simulink model "Citation_2017a"  (R2017a)
settings: Solver=ode5  StartTime=0.0  StopTime=inf  FixedStep=0.01  RelTol=1e-3  EnableMultiTasking=on
InitFcn:
  | initcit
values from neighbouring files (symbols this model uses):
  aeroinit = [dp_ini;inicoef('CX0');inicoef('CXa');inicoef('CXa2');inicoef('CXq')     ;inicoef('CXde');inicoef('CY0');inicoef('CYB');inicoef('CYp');inicoef('CYr')     ;inicoef('CYda');inicoef('CYdr');inicoef('CZ0');inicoef('CZa');inicoef('CZq')     ;inicoef('CZde');inicoef('Cl0');inicoef('ClB');inicoef('Clp');inicoef('Clr')     ;inicoef('Clda');inicoef('Cldr');inicoef('Cm0');inicoef('Cma');inicoef('Cmq')     ; ...(+113 chars)    [initcit.m]
  Clda_thresh = 3.410e-2/2    (= 0.01705)    [initcit.m]
  h_l_old = zeros(6,sample_size)    [initcit.m]
  h_m_old = zeros(4,sample_size)    [initcit.m]
  h_n_old = zeros(6,sample_size)    [initcit.m]
  h_X_old = zeros(5,sample_size)    [initcit.m]
  h_Y_old = zeros(6,sample_size)    [initcit.m]
  h_Z_old = zeros(4,sample_size)    [initcit.m]
  I = [massinit(5),0, -massinit(8);0, massinit(6),0;-massinit(8),0, massinit(7)]    [initcit.m]
  p_l = [inicoef('Cl0');inicoef('ClB');inicoef('Clp');inicoef('Clr')     ;inicoef('Clda');inicoef('Cldr')].*ones(6,sample_size)    [initcit.m]
  p_m = [inicoef('Cm0');inicoef('Cma');inicoef('Cmq')     ;inicoef('Cmde')].*ones(4,sample_size)    [initcit.m]
  p_n = [inicoef('Cn0');inicoef('CnB');inicoef('Cnp');inicoef('Cnr')     ;inicoef('Cnda');inicoef('Cndr')].*ones(6,sample_size)    [initcit.m]
  p_X = [inicoef('CX0');inicoef('CXa');inicoef('CXa2');inicoef('CXq')     ;inicoef('CXde')].*ones(5,sample_size)    [initcit.m]
  p_Y = [inicoef('CY0');inicoef('CYB');inicoef('CYp');inicoef('CYr')     ;inicoef('CYda');inicoef('CYdr')].*ones(6,sample_size)    [initcit.m]
  p_Z = [inicoef('CZ0');inicoef('CZa');inicoef('CZq')     ;inicoef('CZde')].*ones(4,sample_size)    [initcit.m]
  Pcov_l = 10000*eye(6)    [initcit.m]
  Pcov_m = 10000*eye(4)    [initcit.m]
  Pcov_n = 10000*eye(6)    [initcit.m]
  Pcov_X = 10000*eye(5)    [initcit.m]
  Pcov_Y = 10000*eye(6)    [initcit.m]
  Pcov_Z = 10000*eye(4)    [initcit.m]
  replay = 0    [initcit.m]
  T0 = 288.15    [rho_test.m]
  timeend = inputsim.data{1}.Values.Time(end)    [initcit.m]
  Vw915 = 0    [initcit.m]
  winddir = 45*(pi/180)    (= 0.785398163397)    [initcit.m]
  x0 = []    [cessnac550_3d_sfnc.m]    (also in sfunxyauto.m)
  y_l = zeros(1,sample_size)    [initcit.m]
  y_l_est_old = zeros(size(y_l))    [initcit.m]
  y_m = zeros(1,sample_size)    [initcit.m]
  y_m_est_old = zeros(size(y_m))    [initcit.m]
  y_n = zeros(1,sample_size)    [initcit.m]
  y_n_est_old = zeros(size(y_n))    [initcit.m]
  y_X = zeros(1,sample_size)    [initcit.m]
  y_X_est_old = zeros(size(y_X))    [initcit.m]
  y_Y = zeros(1,sample_size)    [initcit.m]
  y_Y_est_old = zeros(size(y_Y))    [initcit.m]
  y_Z = zeros(1,sample_size)    [initcit.m]
  y_Z_est_old = zeros(size(y_Z))    [initcit.m]
undefined symbols (not defined in the file or in its folder): chord, cv1, cv2, cv3, cv4, deltagmax1, deltagmax2, deltagmax3, deltagmax4, Deng, ealphag, ealphas, g0, hDME, hGS, kt1, kt2, kt3, lh, massinit, matbuaf, matdaf, matdam, matdbbf, matdeaf, matdgaf, matdqaf, matduaf, matdwaw, matedhr, mateif, matelhr, matemhr, matemv1, matemv2, matemve, matetam, mateuaf, matfaaf, matfaxl, matff, matibaf, matibmh, matipaf, matipmh, matiraf, matiuaf, matiwaf, matlaf, matlam, matleaf, matleam, matlgaf, matlqaf, matluaf, matmaaf, matmaam, matmaf, matmam, matmbbf ... (+74)
undefined symbols (not defined in the file): matibb
libraries: simulink x13, templibrary x6, vrlib x1
(part 6 of 7)

== system Citation_2017a/Cessna Citation 500/Citation model DASMAT/AIRCRAFT MODEL/AFM/Aeromod/SubSystem/model/CYCAL ==
  in_1 : Inport
  Abs : Abs  SaturateOnIntegerOverflow=on
  CY : Sum  Inputs=+++++  SaturateOnIntegerOverflow=on  InputSameDT=on  OutDataTypeStr=Inherit: Same as first input
  CY/ BETA : Sum  SaturateOnIntegerOverflow=on  InputSameDT=on  OutDataTypeStr=Inherit: Same as first input
  CYBAB : Lookup2D  RowIndex=matybab(2:5,1)  ColumnIndex=matybab(1,2:5)  Table=matybab(2:5,2:5)  SaturateOnIntegerOverflow=on  InputSameDT=on
  CYBAF : Lookup2D  RowIndex=matybaf(2:3,1)  ColumnIndex=matybaf(1,2:3)  Table=matybaf(2:3,2:3)  SaturateOnIntegerOverflow=on  InputSameDT=on
  CYBETA : Product  SaturateOnIntegerOverflow=on  InputSameDT=on  OutDataTypeStr=Inherit: Same as first input
  CYBUAF : Lookup2D  RowIndex=matbuaf(2:3,1)  ColumnIndex=matbuaf(1,2:3)  Table=matbuaf(2:3,2:3)  SaturateOnIntegerOverflow=on  InputSameDT=on
  CYBUC : Product  SaturateOnIntegerOverflow=on  InputSameDT=on  OutDataTypeStr=Inherit: Same as first input
  CYDA : Product  SaturateOnIntegerOverflow=on  InputSameDT=on  OutDataTypeStr=Inherit: Same as first input
  CYDR : Product  Inputs=3  SaturateOnIntegerOverflow=on  InputSameDT=on  OutDataTypeStr=Inherit: Same as first input
  CYGUST : Mux  Inputs=8
  CYR : Product  SaturateOnIntegerOverflow=on  InputSameDT=on  OutDataTypeStr=Inherit: Same as first input
  CYRAF : Lookup2D  RowIndex=matyraf(2:3,1)  ColumnIndex=matyraf(1,2:3)  Table=matyraf(2:3,2:3)  SaturateOnIntegerOverflow=on  InputSameDT=on
  CYRUAF : Lookup2D  RowIndex=matyuaf(2:3,1)  ColumnIndex=matyuaf(1,2:3)  Table=matyuaf(2:3,2:3)  SaturateOnIntegerOverflow=on  InputSameDT=on
  CYWAF : Lookup2D  RowIndex=matywaf(2:3,1)  ColumnIndex=matywaf(1,2:3)  Table=matywaf(2:3,2:3)  SaturateOnIntegerOverflow=on  InputSameDT=on
  Demux : Demux  Outputs=[1 1 1 1 1 1 1 1 1 1 1 1 1 1 1 1 1 1]
  KUUT : Lookup  InputValues=matuut(1,:)  Table=matuut(2,:)  SaturateOnIntegerOverflow=on
  LSFACT : Subsystem
  Prod : Product  SaturateOnIntegerOverflow=on  InputSameDT=on  OutDataTypeStr=Inherit: Same as first input
  Sum : Sum  SaturateOnIntegerOverflow=on  InputSameDT=on  OutDataTypeStr=Inherit: Same as first input
  Terminator_{1..11} (11 alike) : Terminator
  zero : Constant  Value=0
  out_1 : Outport
  out_2 : Outport  Port=2
  wires:
  Demux/18 -> Terminator_11/1
  Demux/17 -> Terminator_10/1
  Demux/16 -> Terminator_9/1
  Demux/13 -> Terminator_8/1
  Demux/12 -> Terminator_7/1
  Demux/11 -> Terminator_6/1
  Demux/8 -> Terminator_5/1
  Demux/7 -> Terminator_4/1
  Demux/6 -> Terminator_3/1
  Demux/2 -> Terminator_2/1
  Demux/1 -> Terminator_1/1
  CY/ BETA/1 -> CYGUST/3
  CYBUAF/1 -> Prod/1
  CYBUC/1 -> CY/5
  CYR/1 -> CY/4
  CYBETA/1 -> CY/1
  CYRAF/1 -> CYR/2
  CYWAF/1 -> CYDA/2
  CYBAB/1 -> Sum/2
  CYBAF/1 -> Sum/1
  Abs/1 -> CYBAB/1
  CY/1 -> out_1/1
  KUUT/1 -> Prod/2
  Demux/14 -> CYBAF/1, CYRUAF/1, CYRAF/1, CYBUAF/1, CYWAF/1
  Demux/5 -> CYBETA/1, Abs/1, CYBUC/1
  Demux/4 -> CYBAF/2, CYWAF/2, CYRAF/2, CYBUAF/2, CYRUAF/2, CYBAB/2
  CYGUST/1 -> out_2/1
  zero/1 -> CYGUST/2, CYGUST/7, CYGUST/8, CYGUST/6, CYGUST/5, CYGUST/4, CYGUST/1
  in_1/1 -> Demux/1
  CYRUAF/1 -> CYDR/2
  Demux/10 -> CYDR/1, LSFACT/1(deltar)
  Sum/1 -> CY/ BETA/1, CYBETA/2
  Prod/1 -> CY/ BETA/2, CYBUC/2
  CYDA/1 -> CY/2
  CYDR/1 -> CY/3
  Demux/3 -> CYR/1
  Demux/15 -> KUUT/1
  Demux/9 -> CYDA/1
  LSFACT/1(LSFACT) -> CYDR/3

== system Citation_2017a/Cessna Citation 500/Citation model DASMAT/AIRCRAFT MODEL/EFM/Engmod/Citation eng_mod/Subsystem1/JT15 Dynamic ==
  In1 : Inport
  Demux : Demux  Outputs=32
  Mux : Mux  Inputs=11
  Subsystem : Subsystem
  Out1 : Outport
  wires:
  Demux/32 -> Subsystem/32(Deng)
  Demux/31 -> Subsystem/31(VIAS)
  Demux/30 -> Subsystem/30(VCAS)
  Demux/29 -> Subsystem/29(VEAS)
  Demux/28 -> Subsystem/28(temptot)
  Demux/27 -> Subsystem/27(ptot)
  Demux/26 -> Subsystem/26(qrel)
  Demux/25 -> Subsystem/25(qc)
  Demux/24 -> Subsystem/24(Reynl)
  Demux/23 -> Subsystem/23(qdyn)
  Demux/22 -> Subsystem/22(Mach)
  Demux/21 -> Subsystem/21(Vsound)
  Demux/20 -> Subsystem/20(Hgeopot)
  Demux/19 -> Subsystem/19(hradio)
  Demux/18 -> Subsystem/18(hpress)
  Demux/17 -> Subsystem/17(grav)
  Demux/16 -> Subsystem/16(temp)
  Demux/15 -> Subsystem/15(rho)
  Demux/14 -> Subsystem/14(pstat)
  Demux/13 -> Subsystem/13(ut)
  Demux/12 -> Subsystem/12(ye)
  Demux/11 -> Subsystem/11(xe)
  Demux/10 -> Subsystem/10(he)
  Demux/9 -> Subsystem/9(psi)
  Demux/8 -> Subsystem/8(theta)
  Demux/7 -> Subsystem/7(phi)
  Demux/6 -> Subsystem/6(beta)
  Demux/5 -> Subsystem/5(alpha)
  Demux/4 -> Subsystem/4(VTAS)
  Demux/3 -> Subsystem/3(rbody)
  Demux/2 -> Subsystem/2(qbody)
  Demux/1 -> Subsystem/1(pbody)
  Subsystem/2(FF) -> Mux/2
  Subsystem/3(N1) -> Mux/3
  Subsystem/4(N2) -> Mux/4
  Subsystem/5(N1c) -> Mux/5
  Subsystem/6(N2c) -> Mux/6
  Subsystem/7(WT) -> Mux/7
  Subsystem/8(ITT) -> Mux/8
  Subsystem/9(EGT) -> Mux/9
  Subsystem/10(OILT) -> Mux/10
  Subsystem/11(OILP) -> Mux/11
  Subsystem/1(Tn) -> Mux/1
  In1/1 -> Demux/1
  Mux/1 -> Out1/1

== system Citation_2017a/Cessna Citation 500/Citation model DASMAT/AIRCRAFT MODEL/EFM/Engmod/Citation eng_mod/Subsystem1/JT15 Dynamic1 ==
  In1 : Inport
  Demux : Demux  Outputs=32
  Mux : Mux  Inputs=11
  Subsystem : Subsystem
  Out1 : Outport
  wires:
  Demux/32 -> Subsystem/32(Deng)
  Demux/31 -> Subsystem/31(VIAS)
  Demux/30 -> Subsystem/30(VCAS)
  Demux/29 -> Subsystem/29(VEAS)
  Demux/28 -> Subsystem/28(temptot)
  Demux/27 -> Subsystem/27(ptot)
  Demux/26 -> Subsystem/26(qrel)
  Demux/25 -> Subsystem/25(qc)
  Demux/24 -> Subsystem/24(Reynl)
  Demux/23 -> Subsystem/23(qdyn)
  Demux/22 -> Subsystem/22(Mach)
  Demux/21 -> Subsystem/21(Vsound)
  Demux/20 -> Subsystem/20(Hgeopot)
  Demux/19 -> Subsystem/19(hradio)
  Demux/18 -> Subsystem/18(hpress)
  Demux/17 -> Subsystem/17(grav)
  Demux/16 -> Subsystem/16(temp)
  Demux/15 -> Subsystem/15(rho)
  Demux/14 -> Subsystem/14(pstat)
  Demux/13 -> Subsystem/13(ut)
  Demux/12 -> Subsystem/12(ye)
  Demux/11 -> Subsystem/11(xe)
  Demux/10 -> Subsystem/10(he)
  Demux/9 -> Subsystem/9(psi)
  Demux/8 -> Subsystem/8(theta)
  Demux/7 -> Subsystem/7(phi)
  Demux/6 -> Subsystem/6(beta)
  Demux/5 -> Subsystem/5(alpha)
  Demux/4 -> Subsystem/4(VTAS)
  Demux/3 -> Subsystem/3(rbody)
  Demux/2 -> Subsystem/2(qbody)
  Demux/1 -> Subsystem/1(pbody)
  Subsystem/2(FF) -> Mux/2
  Subsystem/3(N1) -> Mux/3
  Subsystem/4(N2) -> Mux/4
  Subsystem/5(N1c) -> Mux/5
  Subsystem/6(N2c) -> Mux/6
  Subsystem/7(WT) -> Mux/7
  Subsystem/8(ITT) -> Mux/8
  Subsystem/9(EGT) -> Mux/9
  Subsystem/10(OILT) -> Mux/10
  Subsystem/11(OILP) -> Mux/11
  Subsystem/1(Tn) -> Mux/1
  In1/1 -> Demux/1
  Mux/1 -> Out1/1

== system Citation_2017a/Cessna Citation 500/Citation model DASMAT/AIRCRAFT MODEL/AFM/Aeromod/SubSystem/model/CDCAL/KBASD ==
  hcg : Inport
  deltaf : Inport  Port=2
  VEAS : Inport  Port=3
  Constant : Constant
  Fcn : Fcn  Expr=0.2-u[1]
  Fcn1 : Fcn  Expr=u[2]*(u[1]*180/pi-15)*0.04*(100-u[3])/30
  Fcn2 : Fcn  Expr=1-0.6*u[1]
  KGEDHR : Lookup  InputValues=matedhr(1,:)  Table=matedhr(2,:)  SaturateOnIntegerOverflow=on
  Mux : Mux  Inputs=3
  Sat : Saturate  UpperLimit=1  LowerLimit=0
  Switch : Switch  SaturateOnIntegerOverflow=on  InputSameDT=on
  KBASD : Outport
  wires:
  KGEDHR/1 -> Mux/2
  deltaf/1 -> Mux/1, Fcn/1
  Fcn/1 -> Switch/2
  Constant/1 -> Switch/1
  Switch/1 -> KBASD/1
  VEAS/1 -> Mux/3
  hcg/1 -> KGEDHR/1
  Mux/1 -> Fcn1/1
  Sat/1 -> Fcn2/1
  Fcn1/1 -> Sat/1
  Fcn2/1 -> Switch/3

== system Citation_2017a/Cessna Citation 500/Citation model DASMAT/AIRCRAFT MODEL/AFM/Aeromod/SubSystem/model/CLCAL/CLGEAF ==
  alpha : Inport
  deltaf : Inport  Port=2
  Prod : Product  SaturateOnIntegerOverflow=on  InputSameDT=on  OutDataTypeStr=Inherit: Same as first input
  Sat : Saturate  UpperLimit=0.04  LowerLimit=-inf
  Sum : Sum  SaturateOnIntegerOverflow=on  InputSameDT=on  OutDataTypeStr=Inherit: Same as first input
  VDOMMYR37 : Lookup  InputValues=vdommyr37(1,:)  Table=vdommyr37(2,:)  SaturateOnIntegerOverflow=on
  VDOMMYR40 : Gain  Gain=1.6  SaturateOnIntegerOverflow=on  OutDataTypeStr=Inherit: Same as input  ParamDataTypeStr=Inherit: Same as input
  rad2deg : Gain  Gain=(180/pi)  SaturateOnIntegerOverflow=on  OutDataTypeStr=Inherit: Same as input  ParamDataTypeStr=Inherit: Same as input
  CLGEAF : Outport
  wires:
  VDOMMYR37/1 -> VDOMMYR40/1, Prod/2
  rad2deg/1 -> Prod/1
  Sat/1 -> rad2deg/1
  alpha/1 -> Sat/1
  deltaf/1 -> VDOMMYR37/1
  VDOMMYR40/1 -> Sum/2
  Prod/1 -> Sum/1
  Sum/1 -> CLGEAF/1

== system Citation_2017a/Cessna Citation 500/Citation model DASMAT/AIRCRAFT MODEL/AFM/Aeromod/SubSystem/model/CLCAL/SP0 ==
  deltae : Inport
  Abs : Abs  SaturateOnIntegerOverflow=on
  Fcn : Fcn  Expr=(0.087+0.25*(u[1]-0.087))/(u[1]+1e-11)
  Prod : Product  SaturateOnIntegerOverflow=on  InputSameDT=on  OutDataTypeStr=Inherit: Same as first input
  Sat : Saturate  UpperLimit=1  LowerLimit=-inf
  SP0 : Outport
  wires:
  deltae/1 -> Prod/1, Abs/1
  Sat/1 -> Prod/2
  Fcn/1 -> Sat/1
  Abs/1 -> Fcn/1
  Prod/1 -> SP0/1

== system Citation_2017a/Cessna Citation 500/Citation model DASMAT/AIRCRAFT MODEL/AFM/Aeromod/SubSystem/model/CLLCAL/CIBAB ==
  note: 02-11-2000
      | Modified by A. R. Veldhuijzen
      | sftable3.m was replaced with table3.dll
      | X and Y are exchanged in this Mathworks implementation
  x0 : Inport
  y0 : Inport  Port=2
  z0 : Inport  Port=3
  Mux : Mux  Inputs=3
  S-function : S-Function  FunctionName=table3  Parameters=yindex, xindex ,zindex, table  SFunctionDeploymentMode=off  EnableBusSupport=off
  out_1 : Outport
  wires:
  z0/1 -> Mux/3
  y0/1 -> Mux/1
  x0/1 -> Mux/2
  Mux/1 -> S-function/1
  S-function/1 -> out_1/1

== system Citation_2017a/Cessna Citation 500/Citation model DASMAT/AIRCRAFT MODEL/AFM/Aeromod/SubSystem/model/CLLCAL/LFACT ==
  hcg : Inport
  Sat : Saturate  UpperLimit=1  LowerLimit=0
  hrunway : Fcn  Expr=1-(u[1]-1)/30
  LFACT : Outport
  wires:
  Sat/1 -> LFACT/1
  hcg/1 -> hrunway/1
  hrunway/1 -> Sat/1

== system Citation_2017a/Cessna Citation 500/Citation model DASMAT/AIRCRAFT MODEL/AFM/Aeromod/SubSystem/model/CMCAL/EALPHA ==
  alpha : Inport
  deltaf : Inport  Port=2
  Fcn : Fcn  Expr=1-u[1]*u[2]
  Mux : Mux  Inputs=2
  Sat : Saturate  UpperLimit=1  LowerLimit=0
  Sum : Sum  Inputs=+-  SaturateOnIntegerOverflow=on  InputSameDT=on  OutDataTypeStr=Inherit: Same as first input
  ealphag : Lookup  InputValues=ealphag(1,:)  Table=ealphag(2,:)  SaturateOnIntegerOverflow=on
  ealphas : Lookup  InputValues=ealphas(1,:)  Table=ealphas(2,:)  SaturateOnIntegerOverflow=on
  EALPHA : Outport
  wires:
  deltaf/1 -> ealphag/1, ealphas/1
  alpha/1 -> Sum/1
  Mux/1 -> Fcn/1
  ealphag/1 -> Mux/2
  ealphas/1 -> Sum/2
  Sum/1 -> Mux/1
  Fcn/1 -> Sat/1
  Sat/1 -> EALPHA/1

== system Citation_2017a/Cessna Citation 500/Citation model DASMAT/AIRCRAFT MODEL/AFM/Aeromod/SubSystem/model/CMCAL/LFCMEGAF ==
  alpha : Inport
  Abs : Abs  SaturateOnIntegerOverflow=on
  Fcn : Fcn  Expr=1-5*u[1]
  Neg : Gain  Gain=-1  SaturateOnIntegerOverflow=on  OutDataTypeStr=Inherit: Same as input  ParamDataTypeStr=Inherit: Same as input
  Sat : Saturate  UpperLimit=inf  LowerLimit=0.25
  LFCMEGAF : Outport
  wires:
  Fcn/1 -> Sat/1
  alpha/1 -> Abs/1
  Abs/1 -> Fcn/1
  Sat/1 -> Neg/1
  Neg/1 -> LFCMEGAF/1

== system Citation_2017a/Cessna Citation 500/Citation model DASMAT/AIRCRAFT MODEL/AFM/Aeromod/SubSystem/model/CYCAL/LSFACT ==
  deltar : Inport
  Abs : Abs  SaturateOnIntegerOverflow=on
  Fcn : Fcn  Expr=0.06981/u[1]+2*(u[1]-0.06981)
  Sat : Saturate  UpperLimit=inf  LowerLimit=0.06981
  LSFACT : Outport
  wires:
  deltar/1 -> Abs/1
  Abs/1 -> Sat/1
  Sat/1 -> Fcn/1
  Fcn/1 -> LSFACT/1

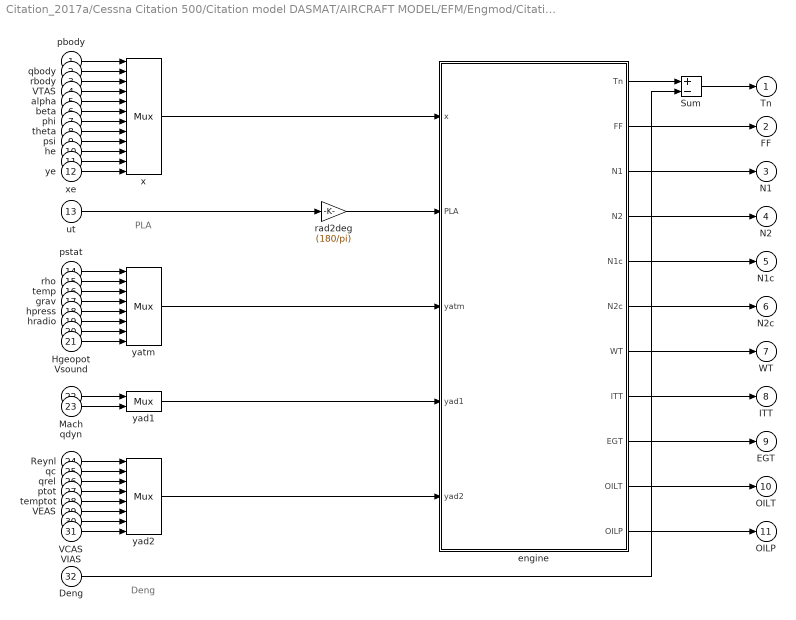
== system Citation_2017a/Cessna Citation 500/Citation model DASMAT/AIRCRAFT MODEL/EFM/Engmod/Citation eng_mod/Subsystem1/JT15 Dynamic/Subsystem ==
  note: Deng
  note: PLA
  pbody : Inport
  qbody : Inport  Port=2
  rbody : Inport  Port=3
  VTAS : Inport  Port=4
  alpha : Inport  Port=5
  beta : Inport  Port=6
  phi : Inport  Port=7
  theta : Inport  Port=8
  psi : Inport  Port=9
  he : Inport  Port=10
  xe : Inport  Port=11
  ye : Inport  Port=12
  ut : Inport  Port=13
  pstat : Inport  Port=14
  rho : Inport  Port=15
  temp : Inport  Port=16
  grav : Inport  Port=17
  hpress : Inport  Port=18
  hradio : Inport  Port=19
  Hgeopot : Inport  Port=20
  Vsound : Inport  Port=21
  Mach : Inport  Port=22
  qdyn : Inport  Port=23
  Reynl : Inport  Port=24
  qc : Inport  Port=25
  qrel : Inport  Port=26
  ptot : Inport  Port=27
  temptot : Inport  Port=28
  VEAS : Inport  Port=29
  VCAS : Inport  Port=30
  VIAS : Inport  Port=31
  Deng : Inport  Port=32
  Sum : Sum  Inputs=+-  SaturateOnIntegerOverflow=on  InputSameDT=on  OutDataTypeStr=Inherit: Same as first input
  engine : Subsystem
  rad2deg : Gain  Gain=(180/pi)  SaturateOnIntegerOverflow=on  OutDataTypeStr=Inherit: Same as input  ParamDataTypeStr=Inherit: Same as input
  x : Mux  Inputs=12
  yad1 : Mux  Inputs=2
  yad2 : Mux  Inputs=8
  yatm : Mux  Inputs=8
  Tn : Outport
  FF : Outport  Port=2
  N1 : Outport  Port=3
  N2 : Outport  Port=4
  N1c : Outport  Port=5
  N2c : Outport  Port=6
  WT : Outport  Port=7
  ITT : Outport  Port=8
  EGT : Outport  Port=9
  OILT : Outport  Port=10
  OILP : Outport  Port=11
  wires:
  Deng/1 -> Sum/2
  engine/1(Tn) -> Sum/1
  Sum/1 -> Tn/1
  Vsound/1 -> yatm/8
  engine/11(OILP) -> OILP/1
  engine/10(OILT) -> OILT/1
  rad2deg/1 -> engine/2(PLA)
  ut/1 -> rad2deg/1
  engine/9(EGT) -> EGT/1
  engine/8(ITT) -> ITT/1
  engine/7(WT) -> WT/1
  engine/6(N2c) -> N2c/1
  engine/5(N1c) -> N1c/1
  engine/4(N2) -> N2/1
  engine/3(N1) -> N1/1
  engine/2(FF) -> FF/1
  yad1/1 -> engine/4(yad1)
  yatm/1 -> engine/3(yatm)
  yad2/1 -> engine/5(yad2)
  qdyn/1 -> yad1/2
  Mach/1 -> yad1/1
  Reynl/1 -> yad2/1
  qc/1 -> yad2/2
  VCAS/1 -> yad2/7
  temptot/1 -> yad2/5
  qrel/1 -> yad2/3
  VIAS/1 -> yad2/8
  VEAS/1 -> yad2/6
  ptot/1 -> yad2/4
  ye/1 -> x/12
  xe/1 -> x/11
  he/1 -> x/10
  psi/1 -> x/9
  VTAS/1 -> x/4
  beta/1 -> x/6
  theta/1 -> x/8
  rbody/1 -> x/3
  alpha/1 -> x/5
  phi/1 -> x/7
  qbody/1 -> x/2
  pbody/1 -> x/1
  pstat/1 -> yatm/1
  rho/1 -> yatm/2
  Hgeopot/1 -> yatm/7
  hpress/1 -> yatm/5
  temp/1 -> yatm/3
  hradio/1 -> yatm/6
  grav/1 -> yatm/4
  x/1 -> engine/1(x)

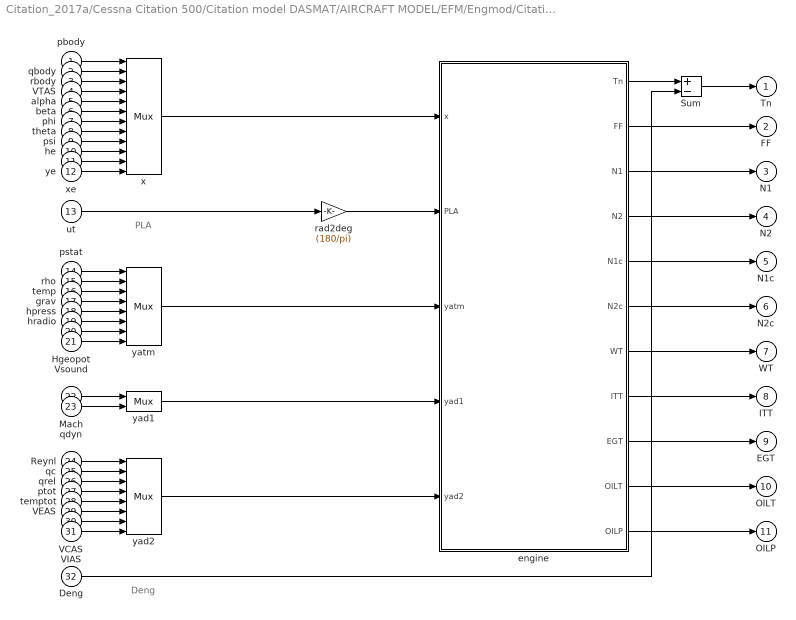
== system Citation_2017a/Cessna Citation 500/Citation model DASMAT/AIRCRAFT MODEL/EFM/Engmod/Citation eng_mod/Subsystem1/JT15 Dynamic1/Subsystem ==
  note: Deng
  note: PLA
  pbody : Inport
  qbody : Inport  Port=2
  rbody : Inport  Port=3
  VTAS : Inport  Port=4
  alpha : Inport  Port=5
  beta : Inport  Port=6
  phi : Inport  Port=7
  theta : Inport  Port=8
  psi : Inport  Port=9
  he : Inport  Port=10
  xe : Inport  Port=11
  ye : Inport  Port=12
  ut : Inport  Port=13
  pstat : Inport  Port=14
  rho : Inport  Port=15
  temp : Inport  Port=16
  grav : Inport  Port=17
  hpress : Inport  Port=18
  hradio : Inport  Port=19
  Hgeopot : Inport  Port=20
  Vsound : Inport  Port=21
  Mach : Inport  Port=22
  qdyn : Inport  Port=23
  Reynl : Inport  Port=24
  qc : Inport  Port=25
  qrel : Inport  Port=26
  ptot : Inport  Port=27
  temptot : Inport  Port=28
  VEAS : Inport  Port=29
  VCAS : Inport  Port=30
  VIAS : Inport  Port=31
  Deng : Inport  Port=32
  Sum : Sum  Inputs=+-  SaturateOnIntegerOverflow=on  InputSameDT=on  OutDataTypeStr=Inherit: Same as first input
  engine : Subsystem
  rad2deg : Gain  Gain=(180/pi)  SaturateOnIntegerOverflow=on  OutDataTypeStr=Inherit: Same as input  ParamDataTypeStr=Inherit: Same as input
  x : Mux  Inputs=12
  yad1 : Mux  Inputs=2
  yad2 : Mux  Inputs=8
  yatm : Mux  Inputs=8
  Tn : Outport
  FF : Outport  Port=2
  N1 : Outport  Port=3
  N2 : Outport  Port=4
  N1c : Outport  Port=5
  N2c : Outport  Port=6
  WT : Outport  Port=7
  ITT : Outport  Port=8
  EGT : Outport  Port=9
  OILT : Outport  Port=10
  OILP : Outport  Port=11
  wires:
  Deng/1 -> Sum/2
  engine/1(Tn) -> Sum/1
  Sum/1 -> Tn/1
  Vsound/1 -> yatm/8
  engine/11(OILP) -> OILP/1
  engine/10(OILT) -> OILT/1
  rad2deg/1 -> engine/2(PLA)
  ut/1 -> rad2deg/1
  engine/9(EGT) -> EGT/1
  engine/8(ITT) -> ITT/1
  engine/7(WT) -> WT/1
  engine/6(N2c) -> N2c/1
  engine/5(N1c) -> N1c/1
  engine/4(N2) -> N2/1
  engine/3(N1) -> N1/1
  engine/2(FF) -> FF/1
  yad1/1 -> engine/4(yad1)
  yatm/1 -> engine/3(yatm)
  yad2/1 -> engine/5(yad2)
  qdyn/1 -> yad1/2
  Mach/1 -> yad1/1
  Reynl/1 -> yad2/1
  qc/1 -> yad2/2
  VCAS/1 -> yad2/7
  temptot/1 -> yad2/5
  qrel/1 -> yad2/3
  VIAS/1 -> yad2/8
  VEAS/1 -> yad2/6
  ptot/1 -> yad2/4
  ye/1 -> x/12
  xe/1 -> x/11
  he/1 -> x/10
  psi/1 -> x/9
  VTAS/1 -> x/4
  beta/1 -> x/6
  theta/1 -> x/8
  rbody/1 -> x/3
  alpha/1 -> x/5
  phi/1 -> x/7
  qbody/1 -> x/2
  pbody/1 -> x/1
  pstat/1 -> yatm/1
  rho/1 -> yatm/2
  Hgeopot/1 -> yatm/7
  hpress/1 -> yatm/5
  temp/1 -> yatm/3
  hradio/1 -> yatm/6
  grav/1 -> yatm/4
  x/1 -> engine/1(x)

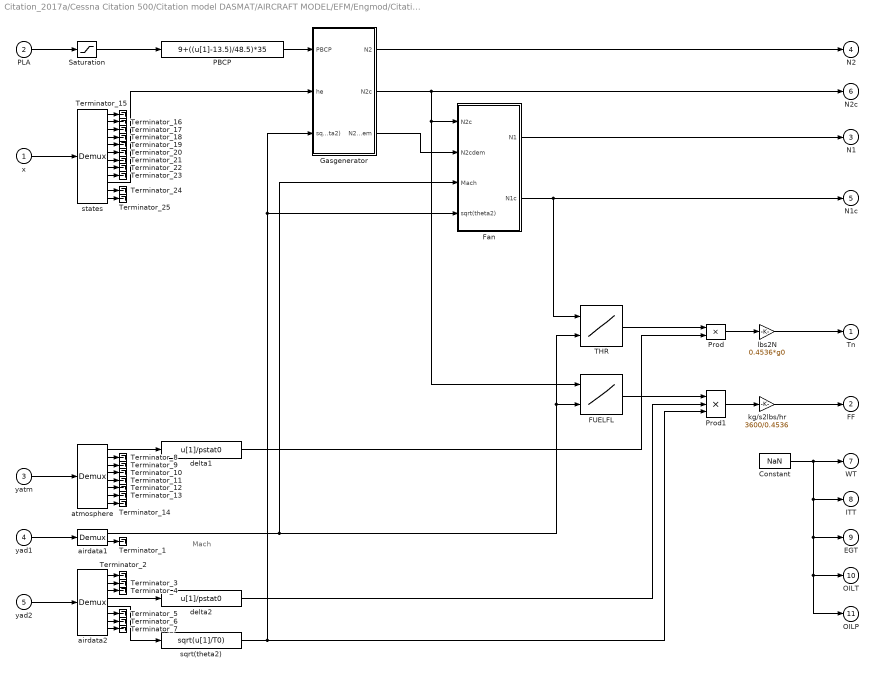
== system Citation_2017a/Cessna Citation 500/Citation model DASMAT/AIRCRAFT MODEL/EFM/Engmod/Citation eng_mod/Subsystem1/JT15 Dynamic/Subsystem/engine ==
  note: Mach
  x : Inport
  PLA : Inport  Port=2
  yatm : Inport  Port=3
  yad1 : Inport  Port=4
  yad2 : Inport  Port=5
  Constant : Constant  Value=NaN
  FUELFL : Lookup2D  RowIndex=matff(2:14,1)  ColumnIndex=matff(1,2:14)  Table=matff(2:14,2:14)  SaturateOnIntegerOverflow=on  InputSameDT=on
  Fan : Subsystem
  Gasgenerator : Subsystem
  PBCP : Fcn  Expr=9+((u[1]-13.5)/48.5)*35
  Prod : Product  SaturateOnIntegerOverflow=on  InputSameDT=on  OutDataTypeStr=Inherit: Same as first input
  Prod1 : Product  Inputs=3  SaturateOnIntegerOverflow=on  InputSameDT=on  OutDataTypeStr=Inherit: Same as first input
  Saturation : Saturate  UpperLimit=62  LowerLimit=13.5
  THR : Lookup2D  RowIndex=matthr(2:12,1)  ColumnIndex=matthr(1,2:12)  Table=matthr(2:12,2:12)  SaturateOnIntegerOverflow=on  InputSameDT=on
  Terminator_{1..25} (25 alike) : Terminator
  airdata1 : Demux  Outputs=2
  airdata2 : Demux  Outputs=8
  atmosphere : Demux  Outputs=8
  delta1 : Fcn  Expr=u[1]/pstat0
  delta2 : Fcn  Expr=u[1]/pstat0
  kg/s2lbs/hr : Gain  Gain=3600/0.4536  SaturateOnIntegerOverflow=on  OutDataTypeStr=Inherit: Same as input  ParamDataTypeStr=Inherit: Same as input
  lbs2N : Gain  Gain=0.4536*g0  SaturateOnIntegerOverflow=on  OutDataTypeStr=Inherit: Same as input  ParamDataTypeStr=Inherit: Same as input
  sqrt(theta2) : Fcn  Expr=sqrt(u[1]/T0)
  states : Demux  Outputs=12
  Tn : Outport
  FF : Outport  Port=2
  N1 : Outport  Port=3
  N2 : Outport  Port=4
  N1c : Outport  Port=5
  N2c : Outport  Port=6
  WT : Outport  Port=7
  ITT : Outport  Port=8
  EGT : Outport  Port=9
  OILT : Outport  Port=10
  OILP : Outport  Port=11
  wires:
  states/12 -> Terminator_25/1
  states/11 -> Terminator_24/1
  states/9 -> Terminator_23/1
  states/8 -> Terminator_22/1
  states/7 -> Terminator_21/1
  states/6 -> Terminator_20/1
  states/5 -> Terminator_19/1
  states/4 -> Terminator_18/1
  states/3 -> Terminator_17/1
  states/2 -> Terminator_16/1
  states/1 -> Terminator_15/1
  atmosphere/8 -> Terminator_14/1
  atmosphere/7 -> Terminator_13/1
  atmosphere/6 -> Terminator_12/1
  atmosphere/5 -> Terminator_11/1
  atmosphere/4 -> Terminator_10/1
  atmosphere/3 -> Terminator_9/1
  atmosphere/2 -> Terminator_8/1
  airdata2/8 -> Terminator_7/1
  airdata2/7 -> Terminator_6/1
  airdata2/6 -> Terminator_5/1
  airdata2/3 -> Terminator_4/1
  airdata2/2 -> Terminator_3/1
  airdata2/1 -> Terminator_2/1
  airdata1/2 -> Terminator_1/1
  Fan/2(N1c) -> THR/1, N1c/1
  Gasgenerator/2(N2c) -> Fan/1(N2c), FUELFL/1, N2c/1
  Gasgenerator/3(N2cdem) -> Fan/2(N2cdem)
  airdata1/1 -> Fan/3(Mach), FUELFL/2, THR/2
  Fan/1(N1) -> N1/1
  sqrt(theta2)/1 -> Fan/4(sqrt(theta2)), Gasgenerator/3(sqrt(theta2)), Prod1/3
  yad2/1 -> airdata2/1
  yad1/1 -> airdata1/1
  yatm/1 -> atmosphere/1
  airdata2/4 -> delta2/1
  airdata2/5 -> sqrt(theta2)/1
  Constant/1 -> ITT/1, EGT/1, OILT/1, OILP/1, WT/1
  Gasgenerator/1(N2) -> N2/1
  delta1/1 -> Prod/2
  Prod/1 -> lbs2N/1
  THR/1 -> Prod/1
  lbs2N/1 -> Tn/1
  states/10 -> Gasgenerator/2(he)
  delta2/1 -> Prod1/2
  atmosphere/1 -> delta1/1
  Prod1/1 -> kg/s2lbs/hr/1
  kg/s2lbs/hr/1 -> FF/1
  Saturation/1 -> PBCP/1
  PLA/1 -> Saturation/1
  x/1 -> states/1
  PBCP/1 -> Gasgenerator/1(PBCP)
  FUELFL/1 -> Prod1/1

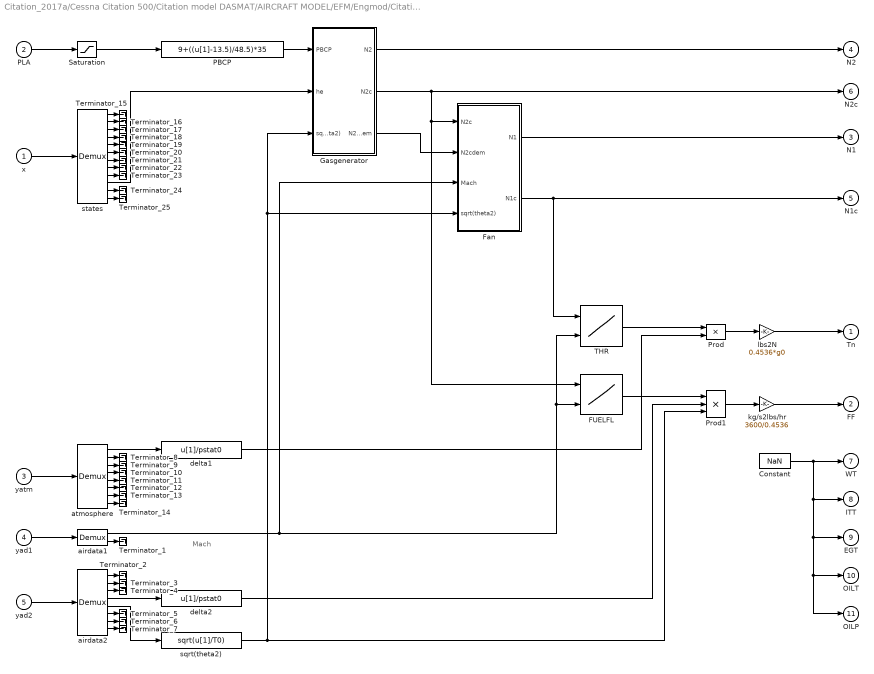
== system Citation_2017a/Cessna Citation 500/Citation model DASMAT/AIRCRAFT MODEL/EFM/Engmod/Citation eng_mod/Subsystem1/JT15 Dynamic1/Subsystem/engine ==
  note: Mach
  x : Inport
  PLA : Inport  Port=2
  yatm : Inport  Port=3
  yad1 : Inport  Port=4
  yad2 : Inport  Port=5
  Constant : Constant  Value=NaN
  FUELFL : Lookup2D  RowIndex=matff(2:14,1)  ColumnIndex=matff(1,2:14)  Table=matff(2:14,2:14)  SaturateOnIntegerOverflow=on  InputSameDT=on
  Fan : Subsystem
  Gasgenerator : Subsystem
  PBCP : Fcn  Expr=9+((u[1]-13.5)/48.5)*35
  Prod : Product  SaturateOnIntegerOverflow=on  InputSameDT=on  OutDataTypeStr=Inherit: Same as first input
  Prod1 : Product  Inputs=3  SaturateOnIntegerOverflow=on  InputSameDT=on  OutDataTypeStr=Inherit: Same as first input
  Saturation : Saturate  UpperLimit=62  LowerLimit=13.5
  THR : Lookup2D  RowIndex=matthr(2:12,1)  ColumnIndex=matthr(1,2:12)  Table=matthr(2:12,2:12)  SaturateOnIntegerOverflow=on  InputSameDT=on
  Terminator_{1..25} (25 alike) : Terminator
  airdata1 : Demux  Outputs=2
  airdata2 : Demux  Outputs=8
  atmosphere : Demux  Outputs=8
  delta1 : Fcn  Expr=u[1]/pstat0
  delta2 : Fcn  Expr=u[1]/pstat0
  kg/s2lbs/hr : Gain  Gain=3600/0.4536  SaturateOnIntegerOverflow=on  OutDataTypeStr=Inherit: Same as input  ParamDataTypeStr=Inherit: Same as input
  lbs2N : Gain  Gain=0.4536*g0  SaturateOnIntegerOverflow=on  OutDataTypeStr=Inherit: Same as input  ParamDataTypeStr=Inherit: Same as input
  sqrt(theta2) : Fcn  Expr=sqrt(u[1]/T0)
  states : Demux  Outputs=12
  Tn : Outport
  FF : Outport  Port=2
  N1 : Outport  Port=3
  N2 : Outport  Port=4
  N1c : Outport  Port=5
  N2c : Outport  Port=6
  WT : Outport  Port=7
  ITT : Outport  Port=8
  EGT : Outport  Port=9
  OILT : Outport  Port=10
  OILP : Outport  Port=11
  wires:
  states/12 -> Terminator_25/1
  states/11 -> Terminator_24/1
  states/9 -> Terminator_23/1
  states/8 -> Terminator_22/1
  states/7 -> Terminator_21/1
  states/6 -> Terminator_20/1
  states/5 -> Terminator_19/1
  states/4 -> Terminator_18/1
  states/3 -> Terminator_17/1
  states/2 -> Terminator_16/1
  states/1 -> Terminator_15/1
  atmosphere/8 -> Terminator_14/1
  atmosphere/7 -> Terminator_13/1
  atmosphere/6 -> Terminator_12/1
  atmosphere/5 -> Terminator_11/1
  atmosphere/4 -> Terminator_10/1
  atmosphere/3 -> Terminator_9/1
  atmosphere/2 -> Terminator_8/1
  airdata2/8 -> Terminator_7/1
  airdata2/7 -> Terminator_6/1
  airdata2/6 -> Terminator_5/1
  airdata2/3 -> Terminator_4/1
  airdata2/2 -> Terminator_3/1
  airdata2/1 -> Terminator_2/1
  airdata1/2 -> Terminator_1/1
  Fan/2(N1c) -> THR/1, N1c/1
  Gasgenerator/2(N2c) -> Fan/1(N2c), FUELFL/1, N2c/1
  Gasgenerator/3(N2cdem) -> Fan/2(N2cdem)
  airdata1/1 -> Fan/3(Mach), FUELFL/2, THR/2
  Fan/1(N1) -> N1/1
  sqrt(theta2)/1 -> Fan/4(sqrt(theta2)), Gasgenerator/3(sqrt(theta2)), Prod1/3
  yad2/1 -> airdata2/1
  yad1/1 -> airdata1/1
  yatm/1 -> atmosphere/1
  airdata2/4 -> delta2/1
  airdata2/5 -> sqrt(theta2)/1
  Constant/1 -> ITT/1, EGT/1, OILT/1, OILP/1, WT/1
  Gasgenerator/1(N2) -> N2/1
  delta1/1 -> Prod/2
  Prod/1 -> lbs2N/1
  THR/1 -> Prod/1
  lbs2N/1 -> Tn/1
  states/10 -> Gasgenerator/2(he)
  delta2/1 -> Prod1/2
  atmosphere/1 -> delta1/1
  Prod1/1 -> kg/s2lbs/hr/1
  kg/s2lbs/hr/1 -> FF/1
  Saturation/1 -> PBCP/1
  PLA/1 -> Saturation/1
  x/1 -> states/1
  PBCP/1 -> Gasgenerator/1(PBCP)
  FUELFL/1 -> Prod1/1

== system Citation_2017a/Cessna Citation 500/Citation model DASMAT/AIRCRAFT MODEL/EFM/Engmod/Citation eng_mod/Subsystem1/JT15 Dynamic/Subsystem/engine/Fan ==
  note: N1c feedback
  note: N1cdot
  N2c : Inport
  N2cdem : Inport  Port=2
  Mach : Inport  Port=3
  sqrt(theta2) : Inport  Port=4
  Droop : Gain  Gain=2  SaturateOnIntegerOverflow=on  OutDataTypeStr=Inherit: Same as input  ParamDataTypeStr=Inherit: Same as input
  Max accel : Subsystem  mask(Min Value){}
      mask help:
      | Output is minimum value of inputs.
      | y=min(u1,u2)
      mask Help: The Min block produces as output the minimum value of two scalars or vectors. If the inputs are vectors, the output will be a vector containing the minimum elements of the vectors.
      mask Display: disp('Min')
  Max decel : Subsystem  mask(Max Value){}
      mask help:
      | Output is maximum value of inputs.
      | y=max(u1,u2)
      mask Help: The Max block produces as output the maximum value of two scalars or vectors. If the inputs are vectors, the output will be a vector containing the maximum elements of the vectors.
      mask Display: disp('Max')
  N1 state : Integrator  InitialCondition=xt0(2)
  N1D : Lookup2D  RowIndex=matn1d(2:14,1)  ColumnIndex=matn1d(1,2:14)  Table=matn1d(2:14,2:14)  SaturateOnIntegerOverflow=on  InputSameDT=on
  Prod : Product  SaturateOnIntegerOverflow=on  InputSameDT=on  OutDataTypeStr=Inherit: Same as first input
  Sum : Sum  Inputs=+-  SaturateOnIntegerOverflow=on  InputSameDT=on  OutDataTypeStr=Inherit: Same as first input
  fN1cmax : Lookup  InputValues="[0 25 40 70 94  120]"  Table="[0   0   1   12 14  18]"  SaturateOnIntegerOverflow=on
  fN1cmin : Lookup  InputValues="[25     50   60   94 100]"  Table="[-0.05  -0.05    -1    -30 -28]"  SaturateOnIntegerOverflow=on
  N1 : Outport
  N1c : Outport  Port=2
  wires:
  sqrt(theta2)/1 -> Prod/2
  N1 state/1 -> Prod/1, Sum/2, N1c/1
  N2c/1 -> fN1cmin/1, fN1cmax/1
  Max decel/1(out_1) -> N1 state/1
  N1D/1 -> Sum/1
  Max accel/1(out_1) -> Max decel/1(in_1)
  fN1cmax/1 -> Max accel/2(in_2)
  fN1cmin/1 -> Max decel/2(in_2)
  Sum/1 -> Droop/1
  Droop/1 -> Max accel/1(in_1)
  Mach/1 -> N1D/2
  Prod/1 -> N1/1
  N2cdem/1 -> N1D/1

== system Citation_2017a/Cessna Citation 500/Citation model DASMAT/AIRCRAFT MODEL/EFM/Engmod/Citation eng_mod/Subsystem1/JT15 Dynamic/Subsystem/engine/Gasgenerator ==
  note: N2 feedback
  note: N2dot
  PBCP : Inport
  he : Inport  Port=2
  sqrt(theta2) : Inport  Port=3
  Droop : Lookup  InputValues=[0 100]  Table="[0.1  2]"  SaturateOnIntegerOverflow=on
  Fcn : Fcn  Expr=u[1]/u[2]
  Fcn1 : Fcn  Expr=u[1]/u[2]
  Governor : Product  SaturateOnIntegerOverflow=on  InputSameDT=on  OutDataTypeStr=Inherit: Same as first input
  Max accel : Subsystem  mask(Max Value){}
      mask help:
      | Output is maximum value of inputs.
      | y=max(u1,u2)
      mask Help: The Max block produces as output the maximum value of two scalars or vectors. If the inputs are vectors, the output will be a vector containing the maximum elements of the vectors.
      mask Display: disp('Max')
  Min accel : Subsystem  mask(Min Value){}
      mask help:
      | Output is minimum value of inputs.
      | y=min(u1,u2)
      mask Help: The Min block produces as output the minimum value of two scalars or vectors. If the inputs are vectors, the output will be a vector containing the minimum elements of the vectors.
      mask Display: disp('Min')
  Mux : Mux  Inputs=2
  Mux1 : Mux  Inputs=2
  N2 state : Integrator  InitialCondition=xt0(1)
  N2D : Lookup2D  RowIndex=matn2d(2:10,1)  ColumnIndex=matn2d(1,2:10)  Table=matn2d(2:10,2:10)  SaturateOnIntegerOverflow=on  InputSameDT=on
  Sum : Sum  Inputs=+-  SaturateOnIntegerOverflow=on  InputSameDT=on  OutDataTypeStr=Inherit: Same as first input
  fN2max : Lookup  InputValues=[25 40 70 94]  Table=[0 3 8 10]  SaturateOnIntegerOverflow=on
  fN2min : Lookup  InputValues="[25     50   60   94 100]"  Table="[-0.05  -0.05    -2    -20 -28]"  SaturateOnIntegerOverflow=on
  ft2FL : Gain  Gain=.01  SaturateOnIntegerOverflow=on  OutDataTypeStr=Inherit: Same as input  ParamDataTypeStr=Inherit: Same as input
  m2ft : Gain  Gain=(1/0.3048)  SaturateOnIntegerOverflow=on  OutDataTypeStr=Inherit: Same as input  ParamDataTypeStr=Inherit: Same as input
  N2 : Outport
  N2c : Outport  Port=2
  N2cdem : Outport  Port=3
  wires:
  sqrt(theta2)/1 -> Mux1/2, Mux/2
  N2D/1 -> Mux/1, Droop/1, Sum/1
  Fcn1/1 -> N2c/1
  Fcn/1 -> N2cdem/1
  Mux1/1 -> Fcn1/1
  Mux/1 -> Fcn/1
  Min accel/1(out_1) -> Max accel/1(in_1)
  ft2FL/1 -> N2D/2
  m2ft/1 -> ft2FL/1
  he/1 -> m2ft/1
  N2 state/1 -> Mux1/1, fN2min/1, fN2max/1, Sum/2, N2/1
  fN2max/1 -> Min accel/2(in_2)
  fN2min/1 -> Max accel/2(in_2)
  PBCP/1 -> N2D/1
  Droop/1 -> Governor/1
  Sum/1 -> Governor/2
  Governor/1 -> Min accel/1(in_1)
  Max accel/1(out_1) -> N2 state/1

== system Citation_2017a/Cessna Citation 500/Citation model DASMAT/AIRCRAFT MODEL/EFM/Engmod/Citation eng_mod/Subsystem1/JT15 Dynamic1/Subsystem/engine/Fan ==
  note: N1c feedback
  note: N1cdot
  N2c : Inport
  N2cdem : Inport  Port=2
  Mach : Inport  Port=3
  sqrt(theta2) : Inport  Port=4
  Droop : Gain  Gain=2  SaturateOnIntegerOverflow=on  OutDataTypeStr=Inherit: Same as input  ParamDataTypeStr=Inherit: Same as input
  Max accel : Subsystem  mask(Min Value){}
      mask help:
      | Output is minimum value of inputs.
      | y=min(u1,u2)
      mask Help: The Min block produces as output the minimum value of two scalars or vectors. If the inputs are vectors, the output will be a vector containing the minimum elements of the vectors.
      mask Display: disp('Min')
  Max decel : Subsystem  mask(Max Value){}
      mask help:
      | Output is maximum value of inputs.
      | y=max(u1,u2)
      mask Help: The Max block produces as output the maximum value of two scalars or vectors. If the inputs are vectors, the output will be a vector containing the maximum elements of the vectors.
      mask Display: disp('Max')
  N1 state : Integrator  InitialCondition=xt0(2)
  N1D : Lookup2D  RowIndex=matn1d(2:14,1)  ColumnIndex=matn1d(1,2:14)  Table=matn1d(2:14,2:14)  SaturateOnIntegerOverflow=on  InputSameDT=on
  Prod : Product  SaturateOnIntegerOverflow=on  InputSameDT=on  OutDataTypeStr=Inherit: Same as first input
  Sum : Sum  Inputs=+-  SaturateOnIntegerOverflow=on  InputSameDT=on  OutDataTypeStr=Inherit: Same as first input
  fN1cmax : Lookup  InputValues="[0 25 40 70 94  120]"  Table="[0   0   1   12 14  18]"  SaturateOnIntegerOverflow=on
  fN1cmin : Lookup  InputValues="[25     50   60   94 100]"  Table="[-0.05  -0.05    -1    -30 -28]"  SaturateOnIntegerOverflow=on
  N1 : Outport
  N1c : Outport  Port=2
  wires:
  sqrt(theta2)/1 -> Prod/2
  N1 state/1 -> Prod/1, Sum/2, N1c/1
  N2c/1 -> fN1cmin/1, fN1cmax/1
  Max decel/1(out_1) -> N1 state/1
  N1D/1 -> Sum/1
  Max accel/1(out_1) -> Max decel/1(in_1)
  fN1cmax/1 -> Max accel/2(in_2)
  fN1cmin/1 -> Max decel/2(in_2)
  Sum/1 -> Droop/1
  Droop/1 -> Max accel/1(in_1)
  Mach/1 -> N1D/2
  Prod/1 -> N1/1
  N2cdem/1 -> N1D/1

== system Citation_2017a/Cessna Citation 500/Citation model DASMAT/AIRCRAFT MODEL/EFM/Engmod/Citation eng_mod/Subsystem1/JT15 Dynamic1/Subsystem/engine/Gasgenerator ==
  note: N2 feedback
  note: N2dot
  PBCP : Inport
  he : Inport  Port=2
  sqrt(theta2) : Inport  Port=3
  Droop : Lookup  InputValues=[0 100]  Table="[0.1  2]"  SaturateOnIntegerOverflow=on
  Fcn : Fcn  Expr=u[1]/u[2]
  Fcn1 : Fcn  Expr=u[1]/u[2]
  Governor : Product  SaturateOnIntegerOverflow=on  InputSameDT=on  OutDataTypeStr=Inherit: Same as first input
  Max accel : Subsystem  mask(Max Value){}
      mask help:
      | Output is maximum value of inputs.
      | y=max(u1,u2)
      mask Help: The Max block produces as output the maximum value of two scalars or vectors. If the inputs are vectors, the output will be a vector containing the maximum elements of the vectors.
      mask Display: disp('Max')
  Min accel : Subsystem  mask(Min Value){}
      mask help:
      | Output is minimum value of inputs.
      | y=min(u1,u2)
      mask Help: The Min block produces as output the minimum value of two scalars or vectors. If the inputs are vectors, the output will be a vector containing the minimum elements of the vectors.
      mask Display: disp('Min')
  Mux : Mux  Inputs=2
  Mux1 : Mux  Inputs=2
  N2 state : Integrator  InitialCondition=xt0(1)
  N2D : Lookup2D  RowIndex=matn2d(2:10,1)  ColumnIndex=matn2d(1,2:10)  Table=matn2d(2:10,2:10)  SaturateOnIntegerOverflow=on  InputSameDT=on
  Sum : Sum  Inputs=+-  SaturateOnIntegerOverflow=on  InputSameDT=on  OutDataTypeStr=Inherit: Same as first input
  fN2max : Lookup  InputValues=[25 40 70 94]  Table=[0 3 8 10]  SaturateOnIntegerOverflow=on
  fN2min : Lookup  InputValues="[25     50   60   94 100]"  Table="[-0.05  -0.05    -2    -20 -28]"  SaturateOnIntegerOverflow=on
  ft2FL : Gain  Gain=.01  SaturateOnIntegerOverflow=on  OutDataTypeStr=Inherit: Same as input  ParamDataTypeStr=Inherit: Same as input
  m2ft : Gain  Gain=(1/0.3048)  SaturateOnIntegerOverflow=on  OutDataTypeStr=Inherit: Same as input  ParamDataTypeStr=Inherit: Same as input
  N2 : Outport
  N2c : Outport  Port=2
  N2cdem : Outport  Port=3
  wires:
  sqrt(theta2)/1 -> Mux1/2, Mux/2
  N2D/1 -> Mux/1, Droop/1, Sum/1
  Fcn1/1 -> N2c/1
  Fcn/1 -> N2cdem/1
  Mux1/1 -> Fcn1/1
  Mux/1 -> Fcn/1
  Min accel/1(out_1) -> Max accel/1(in_1)
  ft2FL/1 -> N2D/2
  m2ft/1 -> ft2FL/1
  he/1 -> m2ft/1
  N2 state/1 -> Mux1/1, fN2min/1, fN2max/1, Sum/2, N2/1
  fN2max/1 -> Min accel/2(in_2)
  fN2min/1 -> Max accel/2(in_2)
  PBCP/1 -> N2D/1
  Droop/1 -> Governor/1
  Sum/1 -> Governor/2
  Governor/1 -> Min accel/1(in_1)
  Max accel/1(out_1) -> N2 state/1

== system Citation_2017a/Cessna Citation 500/Citation model DASMAT/AIRCRAFT MODEL/EFM/Engmod/Citation eng_mod/Subsystem1/JT15 Dynamic/Subsystem/engine/Fan/Max accel ==
  in_1 : Inport
  in_2 : Inport  Port=2
  Sum : Sum  Inputs=-+  SaturateOnIntegerOverflow=on  InputSameDT=on  OutDataTypeStr=Inherit: Same as first input
  Switch : Switch  SaturateOnIntegerOverflow=on  InputSameDT=on
  out_1 : Outport
  wires:
  in_1/1 -> Sum/1, Switch/1
  in_2/1 -> Sum/2, Switch/3
  Sum/1 -> Switch/2
  Switch/1 -> out_1/1

== system Citation_2017a/Cessna Citation 500/Citation model DASMAT/AIRCRAFT MODEL/EFM/Engmod/Citation eng_mod/Subsystem1/JT15 Dynamic/Subsystem/engine/Fan/Max decel ==
  in_1 : Inport
  in_2 : Inport  Port=2
  Sum : Sum  Inputs=+-  SaturateOnIntegerOverflow=on  InputSameDT=on  OutDataTypeStr=Inherit: Same as first input
  Switch : Switch  SaturateOnIntegerOverflow=on  InputSameDT=on
  out_1 : Outport
  wires:
  Switch/1 -> out_1/1
  Sum/1 -> Switch/2
  in_2/1 -> Sum/2, Switch/3
  in_1/1 -> Sum/1, Switch/1

== system Citation_2017a/Cessna Citation 500/Citation model DASMAT/AIRCRAFT MODEL/EFM/Engmod/Citation eng_mod/Subsystem1/JT15 Dynamic/Subsystem/engine/Gasgenerator/Max accel ==
  in_1 : Inport
  in_2 : Inport  Port=2
  Sum : Sum  Inputs=+-  SaturateOnIntegerOverflow=on  InputSameDT=on  OutDataTypeStr=Inherit: Same as first input
  Switch : Switch  SaturateOnIntegerOverflow=on  InputSameDT=on
  out_1 : Outport
  wires:
  Switch/1 -> out_1/1
  Sum/1 -> Switch/2
  in_2/1 -> Sum/2, Switch/3
  in_1/1 -> Sum/1, Switch/1

== system Citation_2017a/Cessna Citation 500/Citation model DASMAT/AIRCRAFT MODEL/EFM/Engmod/Citation eng_mod/Subsystem1/JT15 Dynamic/Subsystem/engine/Gasgenerator/Min accel ==
  in_1 : Inport
  in_2 : Inport  Port=2
  Sum : Sum  Inputs=-+  SaturateOnIntegerOverflow=on  InputSameDT=on  OutDataTypeStr=Inherit: Same as first input
  Switch : Switch  SaturateOnIntegerOverflow=on  InputSameDT=on
  out_1 : Outport
  wires:
  in_1/1 -> Sum/1, Switch/1
  in_2/1 -> Sum/2, Switch/3
  Sum/1 -> Switch/2
  Switch/1 -> out_1/1

== system Citation_2017a/Cessna Citation 500/Citation model DASMAT/AIRCRAFT MODEL/EFM/Engmod/Citation eng_mod/Subsystem1/JT15 Dynamic1/Subsystem/engine/Fan/Max accel ==
  in_1 : Inport
  in_2 : Inport  Port=2
  Sum : Sum  Inputs=-+  SaturateOnIntegerOverflow=on  InputSameDT=on  OutDataTypeStr=Inherit: Same as first input
  Switch : Switch  SaturateOnIntegerOverflow=on  InputSameDT=on
  out_1 : Outport
  wires:
  in_1/1 -> Sum/1, Switch/1
  in_2/1 -> Sum/2, Switch/3
  Sum/1 -> Switch/2
  Switch/1 -> out_1/1

== system Citation_2017a/Cessna Citation 500/Citation model DASMAT/AIRCRAFT MODEL/EFM/Engmod/Citation eng_mod/Subsystem1/JT15 Dynamic1/Subsystem/engine/Fan/Max decel ==
  in_1 : Inport
  in_2 : Inport  Port=2
  Sum : Sum  Inputs=+-  SaturateOnIntegerOverflow=on  InputSameDT=on  OutDataTypeStr=Inherit: Same as first input
  Switch : Switch  SaturateOnIntegerOverflow=on  InputSameDT=on
  out_1 : Outport
  wires:
  Switch/1 -> out_1/1
  Sum/1 -> Switch/2
  in_2/1 -> Sum/2, Switch/3
  in_1/1 -> Sum/1, Switch/1

== system Citation_2017a/Cessna Citation 500/Citation model DASMAT/AIRCRAFT MODEL/EFM/Engmod/Citation eng_mod/Subsystem1/JT15 Dynamic1/Subsystem/engine/Gasgenerator/Max accel ==
  in_1 : Inport
  in_2 : Inport  Port=2
  Sum : Sum  Inputs=+-  SaturateOnIntegerOverflow=on  InputSameDT=on  OutDataTypeStr=Inherit: Same as first input
  Switch : Switch  SaturateOnIntegerOverflow=on  InputSameDT=on
  out_1 : Outport
  wires:
  Switch/1 -> out_1/1
  Sum/1 -> Switch/2
  in_2/1 -> Sum/2, Switch/3
  in_1/1 -> Sum/1, Switch/1

== system Citation_2017a/Cessna Citation 500/Citation model DASMAT/AIRCRAFT MODEL/EFM/Engmod/Citation eng_mod/Subsystem1/JT15 Dynamic1/Subsystem/engine/Gasgenerator/Min accel ==
  in_1 : Inport
  in_2 : Inport  Port=2
  Sum : Sum  Inputs=-+  SaturateOnIntegerOverflow=on  InputSameDT=on  OutDataTypeStr=Inherit: Same as first input
  Switch : Switch  SaturateOnIntegerOverflow=on  InputSameDT=on
  out_1 : Outport
  wires:
  in_1/1 -> Sum/1, Switch/1
  in_2/1 -> Sum/2, Switch/3
  Sum/1 -> Switch/2
  Switch/1 -> out_1/1

== matlab function Citation_2017a/Aerodynamic Parameter Estimation/CX/MATLAB Function ==
  data: P_cov input; P_cov output; pk input; y_new input; hk_new input; y_old input; y_est_old input; h_old input; counter input; pk output; y_old output; y_est_old output; h_old output; forget input; counter output; y_est output; y_new output
function [P_cov, pk,y_old,y_est_old,h_old,counter,y_est,y_new] ...
    =LSQ(P_cov,pk,y_new,hk_new,y_old,y_est_old,h_old,counter,forget)
    lambda=forget;
    P=P_cov;
    p=pk(:,1);
    h=hk_new;
    y=y_new;
    Lk=P*h*(1/(h'*P*h+lambda));
    P=(eye(length(P))-Lk*h')*P*(1/lambda);
    
    p=p+Lk*(y-h'*p);   
    P_cov=P;   
    y_est=h'*p;
 
    
    %% Shift value history
    pk=shift(pk,p);
    y_est_old=(shift(y_est_old',y_est'))'; %this array is oriented vertically 
    h_old=shift(h_old,h);
    y_old=(shift(y_old',y_new'))';          %this array is oriented vertically 
    
    
    
    
    %shift array content right and insert new entry 
   
    function array = shift(array,insert)  

        for i=1:(size(array,2)-1)
             j=size(array,2)-i+1;
               array(:,j)=array(:,j-1);
        end
        array(:,1)=insert(:);

    end
%%
counter=counter+1;
end

== matlab function Citation_2017a/Aero Forces & Moments /Calculate Dynamic Pressure/Calculate Air Density ==
  data: state input; rho output
function rho = fcn(state)
h=state(10);
R=287.05;
l=-0.0065;
h0=0;
T0=288.15;
rho_0=1.225;
h_trop=11000;
h_strat=20000;
g=9.80665;
if h<=h_trop
%    T=T0+(h-h0)*l;
   rho=rho_0*(1+l*(h/T0))^(-(g/(R*l))-1);
   
elseif h>h_trop && h<h_strat
   rho_t=rho_0*(1+l*(h_trop/T0))^(-(g/(R*l))-1);
   T_trop=T0+(h_trop-h0)*l;
   rho=rho_t*(exp(-(g/(R*T_trop))*(h-h_trop)));
   
else
    rho=0; % <- not correct,but this altitude will not be reached anyway
    
end



end

== matlab function Citation_2017a/Aerodynamic Parameter Estimation/CY/MATLAB Function ==
  data: P_cov input; P_cov output; pk input; y_new input; hk_new input; y_old input; y_est_old input; h_old input; counter input; pk output; y_old output; y_est_old output; h_old output; forget input; counter output; y_est output; y_new output
function [P_cov, pk,y_old,y_est_old,h_old,counter,y_est,y_new] ...
    =LSQ(P_cov,pk,y_new,hk_new,y_old,y_est_old,h_old,counter,forget)
    lambda=forget;
    P=P_cov;
    p=pk(:,1);
    h=hk_new;
    y=y_new;
    Lk=P*h*(1/(h'*P*h+lambda));
    P=(eye(length(P))-Lk*h')*P*(1/lambda);
    
    p=p+Lk*(y-h'*p);   
    P_cov=P;   
    y_est=h'*p;
 
    
    %% Shift value history
    pk=shift(pk,p);
    y_est_old=(shift(y_est_old',y_est'))'; %this array is oriented vertically 
    h_old=shift(h_old,h);
    y_old=(shift(y_old',y_new'))';          %this array is oriented vertically 
    
    
    
    
    %shift array content right and insert new entry 
   
    function array = shift(array,insert)  

        for i=1:(size(array,2)-1)
             j=size(array,2)-i+1;
               array(:,j)=array(:,j-1);
        end
        array(:,1)=insert(:);

    end
%%
counter=counter+1;
end

== matlab function Citation_2017a/Aerodynamic Parameter Estimation/CZ/MATLAB Function ==
  data: P_cov input; P_cov output; pk input; y_new input; hk_new input; y_old input; y_est_old input; h_old input; counter input; pk output; y_old output; y_est_old output; h_old output; forget input; counter output; y_est output; y_new output
function [P_cov, pk,y_old,y_est_old,h_old,counter,y_est,y_new] ...
    =LSQ(P_cov,pk,y_new,hk_new,y_old,y_est_old,h_old,counter,forget)
    lambda=forget;
    P=P_cov;
    p=pk(:,1);
    h=hk_new;
    y=y_new;
    Lk=P*h*(1/(h'*P*h+lambda));
    P=(eye(length(P))-Lk*h')*P*(1/lambda);
    
    p=p+Lk*(y-h'*p);   
    P_cov=P;   
    y_est=h'*p;
 
    
    %% Shift value history
    pk=shift(pk,p);
    y_est_old=(shift(y_est_old',y_est'))'; %this array is oriented vertically 
    h_old=shift(h_old,h);
    y_old=(shift(y_old',y_new'))';          %this array is oriented vertically 
    
    
    
    
    %shift array content right and insert new entry 
   
    function array = shift(array,insert)  

        for i=1:(size(array,2)-1)
             j=size(array,2)-i+1;
               array(:,j)=array(:,j-1);
        end
        array(:,1)=insert(:);

    end
%%
counter=counter+1;
end

== matlab function Citation_2017a/Aerodynamic Parameter Estimation/Cl/MATLAB Function ==
  data: P_cov input; P_cov output; pk input; y_new input; hk_new input; y_old input; y_est_old input; h_old input; pk output; y_old output; y_est_old output; h_old output; forget input; y_est output
function [P_cov, pk,y_old,y_est_old,h_old,y_est] ...
    =LSQ(P_cov,pk,y_new,hk_new,y_old,y_est_old,h_old,forget)
    lambda=forget;
    P=P_cov;
    p=pk(:,1);
    h=hk_new;
    y=y_new;
    Lk=P*h*(1/(h'*P*h+lambda));
    P=(eye(length(P))-Lk*h')*P*(1/lambda);
    
    p=p+Lk*(y-h'*p);   
    P_cov=P;   
    y_est=h'*p;
 
    
    %% Shift value history
    pk=shift(pk,p);
    y_est_old=(shift(y_est_old',y_est'))'; %this array is oriented vertically 
    h_old=shift(h_old,h);
    y_old=(shift(y_old',y_new'))';          %this array is oriented vertically 
    
    
    
    
    %shift array content right and insert new entry 
   
    function array = shift(array,insert)  

        for i=1:(size(array,2)-1)
             j=size(array,2)-i+1;
               array(:,j)=array(:,j-1);
        end
        array(:,1)=insert(:);

    end
%%
% counter=counter+1;
end

== matlab function Citation_2017a/Aerodynamic Parameter Estimation/Cm/MATLAB Function ==
  data: P_cov input; P_cov output; pk input; y_new input; hk_new input; y_old input; y_est_old input; h_old input; counter input; pk output; y_old output; y_est_old output; h_old output; forget input; counter output; y_est output; y_new output
function [P_cov, pk,y_old,y_est_old,h_old,counter,y_est,y_new] ...
    =LSQ(P_cov,pk,y_new,hk_new,y_old,y_est_old,h_old,counter,forget)
    lambda=forget;
    P=P_cov;
    p=pk(:,1);
    h=hk_new;
    y=y_new;
    Lk=P*h*(1/(h'*P*h+lambda));
    P=(eye(length(P))-Lk*h')*P*(1/lambda);
    
    p=p+Lk*(y-h'*p);   
    P_cov=P;   
    y_est=h'*p;
 
    
    %% Shift value history
    pk=shift(pk,p);
    y_est_old=(shift(y_est_old',y_est'))'; %this array is oriented vertically 
    h_old=shift(h_old,h);
    y_old=(shift(y_old',y_new'))';          %this array is oriented vertically 
    
    
    
    
    %shift array content right and insert new entry 
   
    function array = shift(array,insert)  

        for i=1:(size(array,2)-1)
             j=size(array,2)-i+1;
               array(:,j)=array(:,j-1);
        end
        array(:,1)=insert(:);

    end
%%
counter=counter+1;
end

== matlab function Citation_2017a/Aerodynamic Parameter Estimation/Cn/MATLAB Function ==
  data: P_cov input; P_cov output; pk input; y_new input; hk_new input; y_old input; y_est_old input; h_old input; counter input; pk output; y_old output; y_est_old output; h_old output; forget input; counter output; y_est output; y_new output
function [P_cov, pk,y_old,y_est_old,h_old,counter,y_est,y_new] ...
    =LSQ(P_cov,pk,y_new,hk_new,y_old,y_est_old,h_old,counter,forget)
    lambda=forget;
    P=P_cov;
    p=pk(:,1);
    h=hk_new;
    y=y_new;
    Lk=P*h*(1/(h'*P*h+lambda));
    P=(eye(length(P))-Lk*h')*P*(1/lambda);
    
    p=p+Lk*(y-h'*p);   
    P_cov=P;   
    y_est=h'*p;
 
    
    %% Shift value history
    pk=shift(pk,p);
    y_est_old=(shift(y_est_old',y_est'))'; %this array is oriented vertically 
    h_old=shift(h_old,h);
    y_old=(shift(y_old',y_new'))';          %this array is oriented vertically 
    
    
    
    
    %shift array content right and insert new entry 
   
    function array = shift(array,insert)  

        for i=1:(size(array,2)-1)
             j=size(array,2)-i+1;
               array(:,j)=array(:,j-1);
        end
        array(:,1)=insert(:);

    end
%%
counter=counter+1;
end

== matlab function Citation_2017a/Pilot/button2toggle 5/MATLAB Function ==
  data: u input
function fcn(u)

if u==1
    disp('Failure Activated');
else
    disp('Failure de-activated');
end

== matlab function Citation_2017a/Pilot/button2toggle 7/MATLAB Function ==
  data: u input; x0 parameter
function  fcn(u,x0)

if u==1
    disp('AutoThrottle enabled');
    fprintf('Desired airspeed: %.3f \n', round(x0(4)));
else
    disp('Autothrottle disabled');
end
